simulink model "8pointDFT"  (R2021b)
settings: Solver=VariableStepAuto  StartTime=0.0  StopTime=10.0  RelTol=1e-3
values from neighbouring files (symbols this model uses):
  j = j + 1    [DSPL5_CircConvUseDFTnIDFT.m]
undefined symbols (not defined in the file or in its folder): i
settings Model: Creator=Admin  LastModifiedBy=Admin

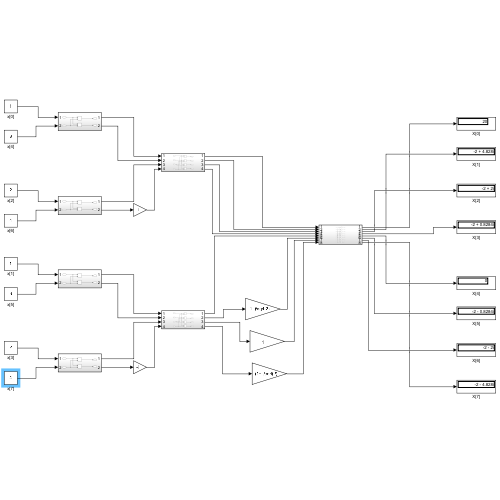
[thumbnail: Simulink's stored preview of the top-level diagram]
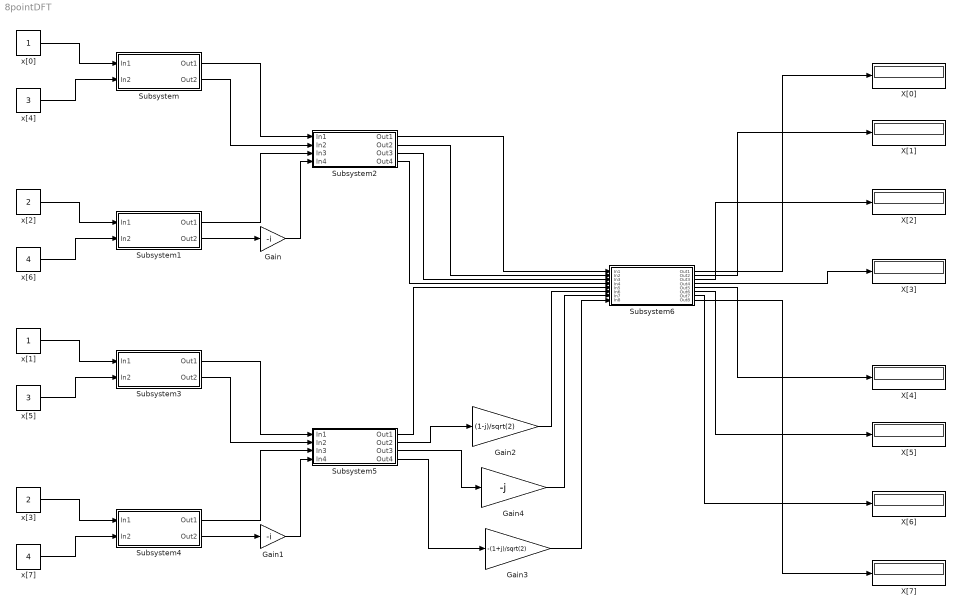
== system 8pointDFT ==
  Gain : Gain  Gain=-i
  Gain1 : Gain  Gain=-i
  Gain2 : Gain  Gain=(1-j)/sqrt(2)
  Gain3 : Gain  Gain=-(1+j)/sqrt(2)
  Gain4 : Gain  Gain=-j
  Subsystem : Subsystem
  Subsystem1 : Subsystem
  Subsystem2 : Subsystem
  Subsystem3 : Subsystem
  Subsystem4 : Subsystem
  Subsystem5 : Subsystem
  Subsystem6 : Subsystem
  X[0] : Display
  X[1] : Display
  X[2] : Display
  X[3] : Display
  X[4] : Display
  X[5] : Display
  X[6] : Display
  X[7] : Display
  x[0] : Constant
  x[1] : Constant
  x[2] : Constant  Value=2
  x[3] : Constant  Value=2
  x[4] : Constant  Value=3
  x[5] : Constant  Value=3
  x[6] : Constant  Value=4
  x[7] : Constant  Value=4
  wires:
  x[0]/1 -> Subsystem/1(In1)
  x[4]/1 -> Subsystem/2(In2)
  x[6]/1 -> Subsystem1/2(In2)
  x[2]/1 -> Subsystem1/1(In1)
  Subsystem/1(Out1) -> Subsystem2/1(In1)
  Subsystem/2(Out2) -> Subsystem2/2(In2)
  Subsystem1/1(Out1) -> Subsystem2/3(In3)
  x[5]/1 -> Subsystem3/2(In2)
  x[1]/1 -> Subsystem3/1(In1)
  x[7]/1 -> Subsystem4/2(In2)
  x[3]/1 -> Subsystem4/1(In1)
  Subsystem1/2(Out2) -> Gain/1
  Gain/1 -> Subsystem2/4(In4)
  Subsystem3/2(Out2) -> Subsystem5/2(In2)
  Subsystem3/1(Out1) -> Subsystem5/1(In1)
  Subsystem4/1(Out1) -> Subsystem5/3(In3)
  Subsystem4/2(Out2) -> Gain1/1
  Gain1/1 -> Subsystem5/4(In4)
  Subsystem5/2(Out2) -> Gain2/1
  Subsystem5/3(Out3) -> Gain4/1
  Subsystem5/4(Out4) -> Gain3/1
  Subsystem6/1(Out1) -> X[0]/1
  Subsystem6/8(Out8) -> X[7]/1
  Subsystem6/2(Out2) -> X[1]/1
  Subsystem6/3(Out3) -> X[2]/1
  Subsystem6/4(Out4) -> X[3]/1
  Subsystem6/5(Out5) -> X[4]/1
  Subsystem6/6(Out6) -> X[5]/1
  Subsystem6/7(Out7) -> X[6]/1
  Gain3/1 -> Subsystem6/8(In8)
  Gain4/1 -> Subsystem6/7(In7)
  Gain2/1 -> Subsystem6/6(In6)
  Subsystem5/1(Out1) -> Subsystem6/5(In5)
  Subsystem2/1(Out1) -> Subsystem6/1(In1)
  Subsystem2/2(Out2) -> Subsystem6/2(In2)
  Subsystem2/3(Out3) -> Subsystem6/3(In3)
  Subsystem2/4(Out4) -> Subsystem6/4(In4)

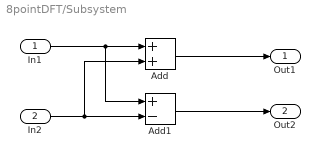
== system 8pointDFT/Subsystem ==
  In1 : Inport
  In2 : Inport  Port=2
  Add : Sum
  Add1 : Sum  Inputs=+-
  Out1 : Outport
  Out2 : Outport  Port=2
  wires:
  In1/1 -> Add1/1, Add/1
  In2/1 -> Add/2, Add1/2
  Add/1 -> Out1/1
  Add1/1 -> Out2/1

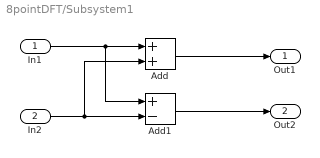
== system 8pointDFT/Subsystem1 ==
  In1 : Inport
  In2 : Inport  Port=2
  Add : Sum
  Add1 : Sum  Inputs=+-
  Out1 : Outport
  Out2 : Outport  Port=2
  wires:
  In1/1 -> Add1/1, Add/1
  In2/1 -> Add/2, Add1/2
  Add/1 -> Out1/1
  Add1/1 -> Out2/1

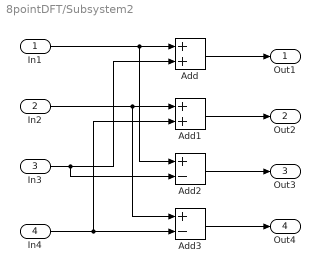
== system 8pointDFT/Subsystem2 ==
  In1 : Inport
  In2 : Inport  Port=2
  In3 : Inport  Port=3
  In4 : Inport  Port=4
  Add : Sum
  Add1 : Sum
  Add2 : Sum  Inputs=+-
  Add3 : Sum  Inputs=+-
  Out1 : Outport
  Out2 : Outport  Port=2
  Out3 : Outport  Port=3
  Out4 : Outport  Port=4
  wires:
  In1/1 -> Add2/1, Add/1
  Add/1 -> Out1/1
  In3/1 -> Add2/2, Add/2
  In2/1 -> Add3/1, Add1/1
  Add1/1 -> Out2/1
  Add3/1 -> Out4/1
  Add2/1 -> Out3/1
  In4/1 -> Add1/2, Add3/2

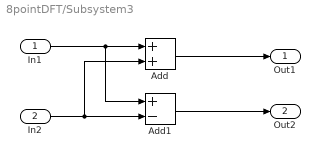
== system 8pointDFT/Subsystem3 ==
  In1 : Inport
  In2 : Inport  Port=2
  Add : Sum
  Add1 : Sum  Inputs=+-
  Out1 : Outport
  Out2 : Outport  Port=2
  wires:
  In1/1 -> Add1/1, Add/1
  In2/1 -> Add/2, Add1/2
  Add/1 -> Out1/1
  Add1/1 -> Out2/1

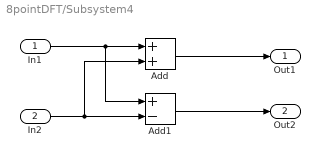
== system 8pointDFT/Subsystem4 ==
  In1 : Inport
  In2 : Inport  Port=2
  Add : Sum
  Add1 : Sum  Inputs=+-
  Out1 : Outport
  Out2 : Outport  Port=2
  wires:
  In1/1 -> Add1/1, Add/1
  In2/1 -> Add/2, Add1/2
  Add/1 -> Out1/1
  Add1/1 -> Out2/1

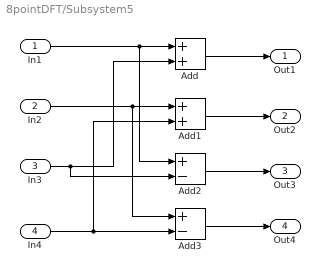
== system 8pointDFT/Subsystem5 ==
  In1 : Inport
  In2 : Inport  Port=2
  In3 : Inport  Port=3
  In4 : Inport  Port=4
  Add : Sum
  Add1 : Sum
  Add2 : Sum  Inputs=+-
  Add3 : Sum  Inputs=+-
  Out1 : Outport
  Out2 : Outport  Port=2
  Out3 : Outport  Port=3
  Out4 : Outport  Port=4
  wires:
  In1/1 -> Add2/1, Add/1
  Add/1 -> Out1/1
  In3/1 -> Add2/2, Add/2
  In2/1 -> Add3/1, Add1/1
  Add1/1 -> Out2/1
  Add3/1 -> Out4/1
  Add2/1 -> Out3/1
  In4/1 -> Add1/2, Add3/2

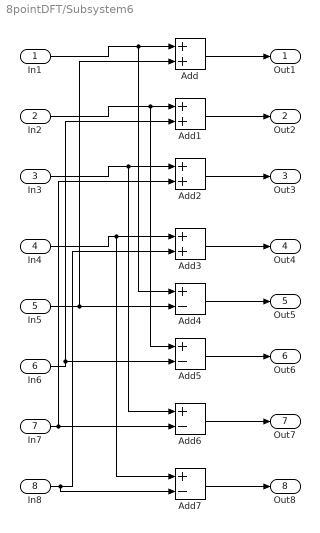
== system 8pointDFT/Subsystem6 ==
  In1 : Inport
  In2 : Inport  Port=2
  In3 : Inport  Port=3
  In4 : Inport  Port=4
  In5 : Inport  Port=5
  In6 : Inport  Port=6
  In7 : Inport  Port=7
  In8 : Inport  Port=8
  Add{,1..3} (4 alike) : Sum
  Add{4..7} (4 alike) : Sum  Inputs=+-
  Out1 : Outport
  Out2 : Outport  Port=2
  Out3 : Outport  Port=3
  Out4 : Outport  Port=4
  Out5 : Outport  Port=5
  Out6 : Outport  Port=6
  Out7 : Outport  Port=7
  Out8 : Outport  Port=8
  wires:
  In1/1 -> Add4/1, Add/1
  In2/1 -> Add5/1, Add1/1
  In3/1 -> Add6/1, Add2/1
  In4/1 -> Add7/1, Add3/1
  In5/1 -> Add4/2, Add/2
  In6/1 -> Add5/2, Add1/2
  In7/1 -> Add6/2, Add2/2
  In8/1 -> Add7/2, Add3/2
  Add/1 -> Out1/1
  Add1/1 -> Out2/1
  Add2/1 -> Out3/1
  Add3/1 -> Out4/1
  Add4/1 -> Out5/1
  Add5/1 -> Out6/1
  Add6/1 -> Out7/1
  Add7/1 -> Out8/1
